simulink model "ODEModelPID"  (R2024a)
settings: Solver=VariableStepAuto  StartTime=0.0  StopTime=simtime  RelTol=1e-9
values from neighbouring files (symbols this model uses):
  A = 4*3.14*0.02^2    (= 0.005024)    [tuneLQR_insilico.m]    (also in tunePID_empirical.m; tunePID_insilico.m)
  alpha = 0.1885    [tuneLQR_insilico.m]    (also in tunePID_empirical.m = 0.19; tunePID_insilico.m)
  beta = 0.6272    [tuneLQR_insilico.m]    (also in tunePID_empirical.m = 0.63; tunePID_insilico.m)
  C_D = 0.47    [tuneLQR_insilico.m]    (also in tunePID_empirical.m; tunePID_insilico.m)
  disturb_magnitude = -7.5    [tuneLQR_insilico.m]    (also in tunePID_insilico.m)
  disturb_time = 20    [tuneLQR_insilico.m]    (also in tunePID_insilico.m)
  g = 9.81    [tuneLQR_insilico.m]    (also in tunePID_empirical.m; tunePID_insilico.m)
  K_D = 30    [tunePID_insilico.m]
  K_F = 5    [tunePID_insilico.m]
  K_I = 10    [tunePID_insilico.m]
  K_P = 300    [tunePID_insilico.m]
  m = 0.00283    [tuneLQR_insilico.m]    (also in tunePID_empirical.m; tunePID_insilico.m)
  noise_sample_time = 0.05    [tuneLQR_insilico.m]    (also in tunePID_empirical.m; tunePID_insilico.m)
  rho = 1.225    [tuneLQR_insilico.m]    (also in tunePID_empirical.m; tunePID_insilico.m)
  steptime = 5    [tuneLQR_insilico.m]    (also in tunePID_empirical.m; tunePID_insilico.m)
  t_d = 0.5    [tuneLQR_insilico.m]    (also in tunePID_empirical.m; tunePID_insilico.m)
  tau = 0.05    [tuneLQR_insilico.m]    (also in tunePID_empirical.m = 0.01; tunePID_insilico.m)
  u_eq = (2*m*g/(rho*A*C_D*alpha^2))^(1/(2*beta))    (= 145.629624466)    [tunePID_empirical.m]    (also in tunePID_insilico.m = 150.797926517)
  z_0 = [0, 0]    [tuneLQR_insilico.m]    (also in tunePID_empirical.m = [0.2, 0]; tunePID_insilico.m)
  z_sp = out.simout(:,2)    [tuneLQR_insilico.m]    (also in tunePID_empirical.m = 0.4; tunePID_insilico.m)
libraries: simulink_extras x1, simulink x1
settings Model: Creator=twallema  LastModifiedBy=twallema
settings SolverCC: AlgebraicLoopSolver=TrustRegion
settings DebuggingCC: UnconnectedInputMsg=warning  UnconnectedOutputMsg=warning  UnconnectedLineMsg=warning
settings ModelReferenceCC: EnableRefExpFcnMdlSchedulingChecks=on
settings SFSimCC: CustomCodeUndefinedFunction=UseInterfaceOnly
settings RTWCC: GPUComputeCapability=3.5

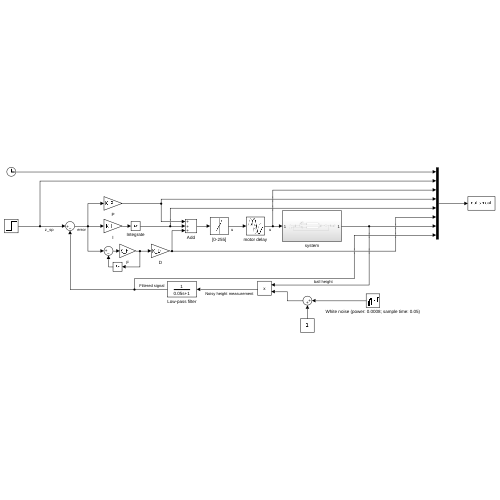
[thumbnail: Simulink's stored preview of the top-level diagram]
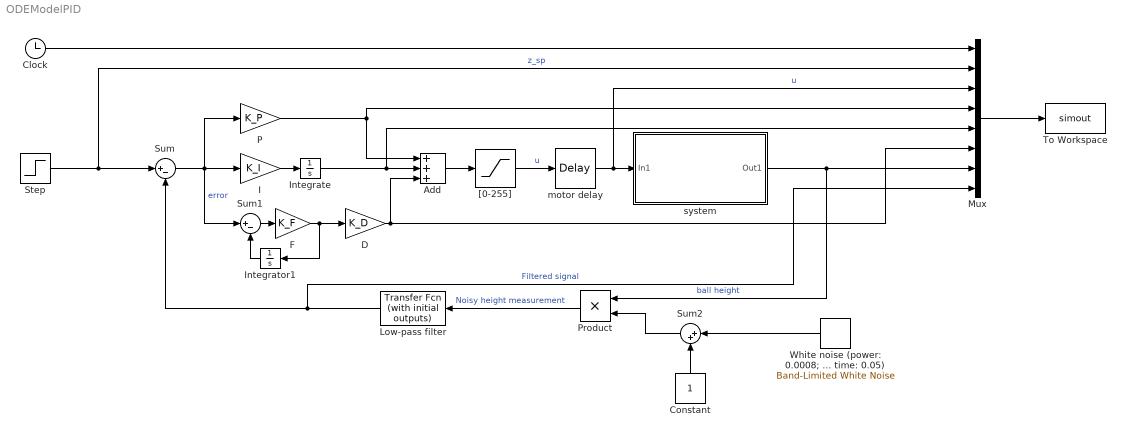
== system ODEModelPID ==
  Add : Sum  Inputs=+++
  Clock : Clock
  Constant : Constant
  D : Gain  Gain=K_D
  F : Gain  Gain=K_F
  I : Gain  Gain=K_I
  Integrate : Integrator  InitialCondition=u_eq
  Integrator1 : Integrator
  Low-pass filter : simulink_extras/Additional Linear/Transfer Fcn (with initial outputs)  N=[1]  D="[tau  1]"  Y0=z_0(1)  U0=z_0(1)
  Mux : Mux  Inputs=8
  P : Gain  Gain=K_P
  Product : Product
  Step : Step  Time=steptime  Before=z_0(1)  After=z_sp  SampleTime=0
  Sum : Sum  Inputs=|+-
  Sum1 : Sum  Inputs=|+-
  Sum2 : Sum  Inputs=|++
  To Workspace : ToWorkspace  VariableName=simout  SampleTime=-1
  White noise (power: 0.0008; sample time: 0.05) : simulink/Sources/Band-Limited White Noise  Cov=noise_power  Ts=noise_sample_time  seed=[23341]
  "[0-255]" : Saturate  UpperLimit=255  LowerLimit=0
  motor delay : TransportDelay  DelayTime=t_d  InitialOutput=u_eq
  system : Subsystem
  wires:
  Mux/1 -> To Workspace/1
  system/1(Out1) -> Product/1, Mux/7  "ball height"
  Sum/1 -> I/1, Sum1/1, P/1  "error"
  motor delay/1 -> Mux/3, system/1(In1)  "u"
  Add/1 -> "[0-255]"/1
  P/1 -> Mux/4, Add/1
  Sum1/1 -> F/1
  Integrator1/1 -> Sum1/2
  D/1 -> Mux/6, Add/3
  Step/1 -> Mux/2, Sum/1  "z_sp"
  Clock/1 -> Mux/1
  F/1 -> D/1, Integrator1/1
  Product/1 -> Low-pass filter/1  "Noisy height measurement"
  White noise (power: 0.0008; sample time: 0.05)/1 -> Sum2/1
  Sum2/1 -> Product/2
  Constant/1 -> Sum2/2
  Low-pass filter/1 -> Sum/2, Mux/8  "Filtered signal"
  I/1 -> Integrate/1
  Integrate/1 -> Mux/5, Add/2
  "[0-255]"/1 -> motor delay/1  "u"

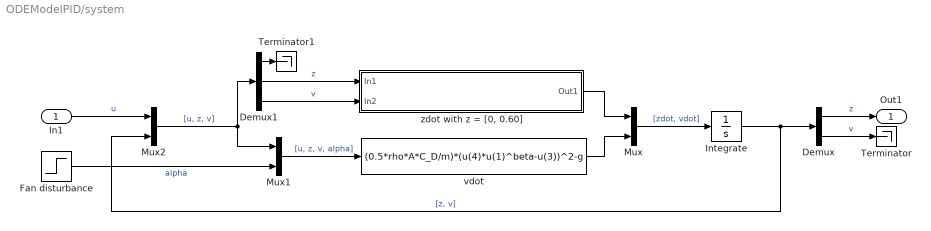
== system ODEModelPID/system ==
  In1 : Inport
  Demux : Demux  Outputs=2
  Demux1 : Demux  Outputs=3
  Fan disturbance : Step  Time=disturb_time  Before=alpha  After=alpha*(1+disturb_magnitude/100)  SampleTime=0
  Integrate : Integrator  InitialCondition=z_0
  Mux : Mux  Inputs=2
  Mux1 : Mux  Inputs=2
  Mux2 : Mux  Inputs=2
  Terminator : Terminator
  Terminator1 : Terminator
  vdot : Fcn  Expr=(0.5*rho*A*C_D/m)*(u(4)*u(1)^beta-u(3))^2-g
  "zdot with z = [0, 0.60]" : Subsystem
  Out1 : Outport  VectorParamsAs1DForOutWhenUnconnected=off
  wires:
  vdot/1 -> Mux/2
  Mux2/1 -> Mux1/1, Demux1/1  "[u, z, v]"
  In1/1 -> Mux2/1  "u"
  Integrate/1 -> Demux/1, Mux2/2  "[z, v]"
  Mux/1 -> Integrate/1  "[zdot, vdot]"
  Demux1/1 -> Terminator1/1
  Demux1/3 -> "zdot with z = [0, 0.60]"/2(In2)  "v"
  Demux1/2 -> "zdot with z = [0, 0.60]"/1(In1)  "z"
  "zdot with z = [0, 0.60]"/1(Out1) -> Mux/1
  Mux1/1 -> vdot/1  "[u, z, v, alpha]"
  Fan disturbance/1 -> Mux1/2  "alpha"
  Demux/1 -> Out1/1  "z"
  Demux/2 -> Terminator/1  "v"

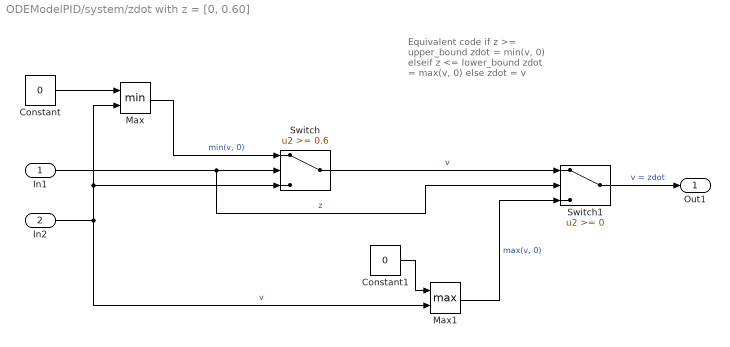
== system ODEModelPID/system/zdot with z = [0, 0.60] ==
  note: Equivalent code
      |
      | if z >= upper_bound
      | zdot = min(v, 0)
      | elseif z <= lower_bound
      | zdot = max(v, 0)
      | else
      | zdot = v
  In1 : Inport
  In2 : Inport  Port=2
  Constant : Constant  Value=0
  Constant1 : Constant  Value=0
  Max : MinMax  Inputs=2
  Max1 : MinMax  Function=max  Inputs=2
  Switch : Switch  Threshold=0.6  SaturateOnIntegerOverflow=off  InputSameDT=off
  Switch1 : Switch  SaturateOnIntegerOverflow=off  InputSameDT=off
  Out1 : Outport
  wires:
  Max1/1 -> Switch1/3  "max(v, 0)"
  Constant/1 -> Max/1
  Constant1/1 -> Max1/1
  Switch/1 -> Switch1/1  "v"
  Max/1 -> Switch/1  "min(v, 0)"
  Switch1/1 -> Out1/1  "v = zdot"
  In1/1 -> Switch/2, Switch1/2  "z"
  In2/1 -> Max/2, Switch/3, Max1/2  "v"
